simulink model "QueuingExecutionBehavior"  (R2015a)
settings: Solver=VariableStepDiscrete  StartTime=0.0  StopTime=1000  RelTol=1e-3
settings Model: Creator=tsprock3  LastModifiedBy=tsprock3

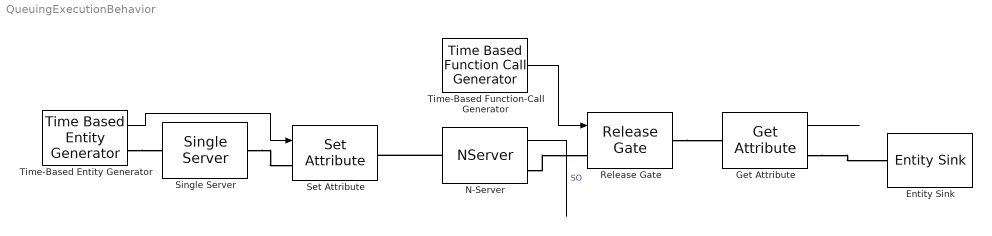
== system QueuingExecutionBehavior ==
  Entity Sink : EntitySink
  Get Attribute : GetAttribute  AttributeName=IndexID  EvaluatedDefaultAttributeValue={ []}
      settings: OutputPortMap=o1
  N-Server : NServer  ServiceTime=0  StatServerOccupancy=on
      settings: OutputPortMap=o7
  Release Gate : ReleaseGate  OpenGateUpon=Function call from port fcn
  Set Attribute : SetAttribute  AttributeName=IndexID  AttributeFrom=Signal port  EvaluatedAttributeValue={ []}
  Single Server : SingleServer  ServiceTime=0
  Time-Based Entity Generator : TimeBasedEntityGenerator  StatNumberDeparted=on
  Time-Based Function-Call Generator : TimeBasedFunctionCallGenerator  Period=1.25
  wires:
  Time-Based Entity Generator/1 -> Set Attribute/1
  Time-Based Function-Call Generator/1 -> Release Gate/1
  Get Attribute/1 -> ?
  N-Server/1 -> ?  "SO"
  connections:
  Time-Based Entity Generator/RConn1 -- Single Server/LConn1
  Single Server/RConn1 -- Set Attribute/LConn1
  N-Server/LConn1 -- Set Attribute/RConn1
  N-Server/RConn1 -- Release Gate/LConn1
  Release Gate/RConn1 -- Get Attribute/LConn1
  Get Attribute/RConn1 -- Entity Sink/LConn1
